simulink model "Milford"  (R2017a)
settings: Solver=FixedStepAuto  StartTime=0.0  StopTime=Cycle_End  FixedStep=0.01  MaxStep=0.01  RelTol=1e-3  EnableMultiTasking=on
PostLoadFcn:
  | , if any(exist('dsrtsu_mdlpostloadfcn', 'file') == [2, 3, 6]), try dsrtsu_mdlpostloadfcn('Execute', bdroot); catch fprintf('Error in PostLoadFcn (dsrtsu_mdlpostloadfcn) for model "%s":\n %s\n', bdroot, lasterr); end, end,
undefined symbols (not defined in the file): Actuators, APP1_OOR, APP2_OOR, APP_Mismatch, Brk_Flt, cal, ClutchEngag, DiscIntNeverNeededParam, eng, Engine, EngOverTemp, ENGTRQ_MSMCH_Degraded_CP, ENGTRQ_MSMCH_ErrCritical_CP, ENGTRQ_MSMCH_LimpHome_CP, EngTrqMismatch, ESSOverTemp, gb, Gearbox, KeyPos_Flt, lib_Actuators, lib_Sensors_2017a, lib_Transmission, Loss, LossCAN, MCUOverTemp, mot, MotDirMismatch, MotOverTemp, MotTrqMismatch, mph2kph, PRNDL_Flt, Ratio, RegenFault, Sensors, Spd, time, Transmission
libraries: simulink x110, powerlib_meascontrol x6, EC2_libraries x5, dspsigops x3, lib_Chassis x1, lib_DCDC x1, lib_Differential x1, lib_HVESS x1, lib_Engine x1, lib_OBC x1, Transmission_Validation x1, lib_Wheels x1
(part 2 of 9)

== system Milford/Fault Trigger /Component Diagnostics setting/Override  ESSOverTemp ==
  note: This subsystem is used to override the model value of a signal to a constant value
  note: Override Switch Subsystem
  In1 : Inport
  Constant : Constant  Value=0
  Multiport Switch : MultiPortSwitch  DataPortOrder=Zero-based contiguous  Inputs=2
  Signal Override Switch 0 = Use Model 1 = Use Constant : Constant  Value=ESSOverTemp_ON
  Out1 : Outport
  wires:
  Signal Override Switch 0 = Use Model 1 = Use Constant/1 -> Multiport Switch/1
  In1/1 -> Multiport Switch/2
  Multiport Switch/1 -> Out1/1
  Constant/1 -> Multiport Switch/3

== system Milford/Fault Trigger /Component Diagnostics setting/Override  EngOverTemp ==
  note: Override Switch Subsystem
  note: This subsystem is used to override the model value of a signal to a constant value
  In1 : Inport
  Constant : Constant  Value=0
  Multiport Switch : MultiPortSwitch  DataPortOrder=Zero-based contiguous  Inputs=2
  Signal Override Switch 0 = Use Model 1 = Use Constant : Constant  Value=EngOverTemp_ON
  Out1 : Outport
  wires:
  Constant/1 -> Multiport Switch/3
  Multiport Switch/1 -> Out1/1
  In1/1 -> Multiport Switch/2
  Signal Override Switch 0 = Use Model 1 = Use Constant/1 -> Multiport Switch/1

== system Milford/Fault Trigger /Component Diagnostics setting/Override  EngTrqMismatch ==
  note: This subsystem is used to override the model value of a signal to a constant value
  note: Override Switch Subsystem
  In1 : Inport
  Constant : Constant  Value=0
  Multiport Switch : MultiPortSwitch  DataPortOrder=Zero-based contiguous  Inputs=2
  Signal Override Switch 0 = Use Model 1 = Use Constant : Constant  Value=EngTrqMismatch_ON
  Out1 : Outport
  wires:
  Signal Override Switch 0 = Use Model 1 = Use Constant/1 -> Multiport Switch/1
  In1/1 -> Multiport Switch/2
  Multiport Switch/1 -> Out1/1
  Constant/1 -> Multiport Switch/3

== system Milford/Fault Trigger /Component Diagnostics setting/Override  LossCAN ==
  note: Override Switch Subsystem
  note: This subsystem is used to override the model value of a signal to a constant value
  In1 : Inport
  Constant : Constant  Value=0
  Multiport Switch : MultiPortSwitch  DataPortOrder=Zero-based contiguous  Inputs=2
  Signal Override Switch 0 = Use Model 1 = Use Constant : Constant  Value=LossCAN_ON
  Out1 : Outport
  wires:
  Constant/1 -> Multiport Switch/3
  Multiport Switch/1 -> Out1/1
  In1/1 -> Multiport Switch/2
  Signal Override Switch 0 = Use Model 1 = Use Constant/1 -> Multiport Switch/1

== system Milford/Fault Trigger /Component Diagnostics setting/Override  MCUOverTemp ==
  note: This subsystem is used to override the model value of a signal to a constant value
  note: Override Switch Subsystem
  In1 : Inport
  Constant : Constant  Value=0
  Multiport Switch : MultiPortSwitch  DataPortOrder=Zero-based contiguous  Inputs=2
  Signal Override Switch 0 = Use Model 1 = Use Constant : Constant  Value=MCUOverTemp_ON
  Out1 : Outport
  wires:
  Signal Override Switch 0 = Use Model 1 = Use Constant/1 -> Multiport Switch/1
  In1/1 -> Multiport Switch/2
  Multiport Switch/1 -> Out1/1
  Constant/1 -> Multiport Switch/3

== system Milford/Fault Trigger /Component Diagnostics setting/Override  MotDirMismatch ==
  note: Override Switch Subsystem
  note: This subsystem is used to override the model value of a signal to a constant value
  In1 : Inport
  Constant : Constant  Value=0
  Multiport Switch : MultiPortSwitch  DataPortOrder=Zero-based contiguous  Inputs=2
  Signal Override Switch 0 = Use Model 1 = Use Constant : Constant  Value=MotDirMismatch_ON
  Out1 : Outport
  wires:
  Constant/1 -> Multiport Switch/3
  Multiport Switch/1 -> Out1/1
  In1/1 -> Multiport Switch/2
  Signal Override Switch 0 = Use Model 1 = Use Constant/1 -> Multiport Switch/1

== system Milford/Fault Trigger /Component Diagnostics setting/Override  MotOverTemp ==
  note: Override Switch Subsystem
  note: This subsystem is used to override the model value of a signal to a constant value
  In1 : Inport
  Constant : Constant  Value=0
  Multiport Switch : MultiPortSwitch  DataPortOrder=Zero-based contiguous  Inputs=2
  Signal Override Switch 0 = Use Model 1 = Use Constant : Constant  Value=MotOverTemp_ON
  Out1 : Outport
  wires:
  Constant/1 -> Multiport Switch/3
  Multiport Switch/1 -> Out1/1
  In1/1 -> Multiport Switch/2
  Signal Override Switch 0 = Use Model 1 = Use Constant/1 -> Multiport Switch/1

== system Milford/Fault Trigger /Component Diagnostics setting/Override  MotTrqMismatch ==
  note: This subsystem is used to override the model value of a signal to a constant value
  note: Override Switch Subsystem
  In1 : Inport
  Constant : Constant  Value=0
  Multiport Switch : MultiPortSwitch  DataPortOrder=Zero-based contiguous  Inputs=2
  Signal Override Switch 0 = Use Model 1 = Use Constant : Constant  Value=MotTrqMismatch_ON
  Out1 : Outport
  wires:
  Signal Override Switch 0 = Use Model 1 = Use Constant/1 -> Multiport Switch/1
  In1/1 -> Multiport Switch/2
  Multiport Switch/1 -> Out1/1
  Constant/1 -> Multiport Switch/3

== system Milford/Fault Trigger /Driver Interface Diagnostics setting/Override  APP1_OOR ==
  note: Signal Override Switch
      | 0 = Use Model
      | 1 = Use Constant
  note: Override Switch Subsystem
  note: This subsystem is used to override the model value of a signal to a constant value
  In1 : Inport
  APP1_OOR_ON : Constant  Value=APP1_OOR_ON
  Constant : Constant  Value=0
  Multiport Switch : MultiPortSwitch  DataPortOrder=Zero-based contiguous  Inputs=2
  Out1 : Outport
  wires:
  Constant/1 -> Multiport Switch/3
  Multiport Switch/1 -> Out1/1
  In1/1 -> Multiport Switch/2
  APP1_OOR_ON/1 -> Multiport Switch/1

== system Milford/Fault Trigger /Driver Interface Diagnostics setting/Override  APP2_OOR ==
  note: Signal Override Switch
      | 0 = Use Model
      | 1 = Use Constant
  note: This subsystem is used to override the model value of a signal to a constant value
  note: Override Switch Subsystem
  In1 : Inport
  APP2_OOR_ON : Constant  Value=APP2_OOR_ON
  Constant : Constant  Value=0
  Multiport Switch : MultiPortSwitch  DataPortOrder=Zero-based contiguous  Inputs=2
  Out1 : Outport
  wires:
  APP2_OOR_ON/1 -> Multiport Switch/1
  In1/1 -> Multiport Switch/2
  Multiport Switch/1 -> Out1/1
  Constant/1 -> Multiport Switch/3

== system Milford/Fault Trigger /Driver Interface Diagnostics setting/Override  APP_Mismatch ==
  note: Signal Override Switch
      | 0 = Use Model
      | 1 = Use Constant
  note: Override Switch Subsystem
  note: This subsystem is used to override the model value of a signal to a constant value
  In1 : Inport
  APP_Mismatch_Override : Constant  Value=Mismatch_APP_ON
  Constant : Constant  Value=0
  Multiport Switch : MultiPortSwitch  DataPortOrder=Zero-based contiguous  Inputs=2
  Out1 : Outport
  wires:
  Constant/1 -> Multiport Switch/3
  Multiport Switch/1 -> Out1/1
  In1/1 -> Multiport Switch/2
  APP_Mismatch_Override/1 -> Multiport Switch/1

== system Milford/Fault Trigger /Driver Interface Diagnostics setting/Override  BPP_Flt ==
  note: Signal Override Switch
      | 0 = Use Model
      | 1 = Use Constant
  note: This subsystem is used to override the model value of a signal to a constant value
  note: Override Switch Subsystem
  In1 : Inport
  Brk_Flt_ON : Constant  Value=Brk_Flt_ON
  Constant : Constant  Value=0
  Multiport Switch : MultiPortSwitch  DataPortOrder=Zero-based contiguous  Inputs=2
  Out1 : Outport
  wires:
  Brk_Flt_ON/1 -> Multiport Switch/1
  In1/1 -> Multiport Switch/2
  Multiport Switch/1 -> Out1/1
  Constant/1 -> Multiport Switch/3

== system Milford/Fault Trigger /Driver Interface Diagnostics setting/Override  KeyPos_Flt ==
  note: Signal Override Switch
      | 0 = Use Model
      | 1 = Use Constant
  note: Override Switch Subsystem
  note: This subsystem is used to override the model value of a signal to a constant value
  In1 : Inport
  Constant : Constant  Value=0
  KeyPos_Flt_ON : Constant  Value=KeyPos_Flt_ON
  Multiport Switch : MultiPortSwitch  DataPortOrder=Zero-based contiguous  Inputs=2
  Out1 : Outport
  wires:
  Constant/1 -> Multiport Switch/3
  Multiport Switch/1 -> Out1/1
  In1/1 -> Multiport Switch/2
  KeyPos_Flt_ON/1 -> Multiport Switch/1

== system Milford/Fault Trigger /Driver Interface Diagnostics setting/Override  PRNDL_Flt ==
  note: Signal Override Switch
      | 0 = Use Model
      | 1 = Use Constant
  note: This subsystem is used to override the model value of a signal to a constant value
  note: Override Switch Subsystem
  In1 : Inport
  Constant : Constant  Value=0
  Multiport Switch : MultiPortSwitch  DataPortOrder=Zero-based contiguous  Inputs=2
  PRNDL_Flt_ON : Constant  Value=PRNDL_Flt_ON
  Out1 : Outport
  wires:
  PRNDL_Flt_ON/1 -> Multiport Switch/1
  In1/1 -> Multiport Switch/2
  Multiport Switch/1 -> Out1/1
  Constant/1 -> Multiport Switch/3

== system Milford/Sensors/CAN/EBCAN ==
  In1 : Inport
  BMS_Antrieb : Subsystem
  Bus Creator : BusCreator  Inputs=3
  Bus Selector : BusSelector  OutputSignals=ECM_CAN,BMS_CAN.BMS_Hybrid
  CCM : Subsystem
  ECM : Subsystem
  Out1 : Outport
  wires:
  Bus Selector/2 -> BMS_Antrieb/1(In1), CCM/1(In1)  "<BMS_Hybrid>"
  Bus Selector/1 -> ECM/1(In1)  "<ECM_CAN>"
  In1/1 -> Bus Selector/1
  CCM/1(Out1) -> Bus Creator/3  "from_CCM"
  Bus Creator/1 -> Out1/1
  BMS_Antrieb/1(Out1) -> Bus Creator/2  "from_BMSAntrieb"
  ECM/1(Out1) -> Bus Creator/1  "from_ECM"

== system Milford/Sensors/CAN/HV_CAN ==
  In1 : Inport
  BMS_Hybrid : Subsystem
  Bus Creator : BusCreator  Inputs=2
  Bus Selector : BusSelector  OutputSignals=BMS_CAN.BMS_Plugin,OBC_CAN
  OBC : Subsystem
  Out1 : Outport
  wires:
  Bus Selector/2 -> OBC/1(In1)  "<OBC_CAN>"
  Bus Selector/1 -> BMS_Hybrid/1(In1)  "<BMS_Plugin>"
  In1/1 -> Bus Selector/1
  Bus Creator/1 -> Out1/1
  OBC/1(Out1) -> Bus Creator/2  "from_OBC"
  BMS_Hybrid/1(Out1) -> Bus Creator/1  "from_BMSHybrid"

== system Milford/Sensors/CAN/VEH_CAN ==
  In1 : Inport
  BCM : Subsystem
  Bus Creator : BusCreator  Inputs=4
  Bus Selector : BusSelector  OutputSignals=TCM_CAN,BCM_CAN
  EBCM : Subsystem  Commented=on
  Ground : Ground  Commented=on
  Ground1 : Ground  Commented=on
  ICCM : Subsystem  Commented=on
  TCM : Subsystem
  Out1 : Outport
  wires:
  Ground/1 -> EBCM/1(In1)  "<EBCM>"
  Ground1/1 -> ICCM/1(In1)  "<ONSTAR>"
  Bus Selector/2 -> BCM/1(In1)  "<BCM_CAN>"
  Bus Selector/1 -> TCM/1(In1)  "<TCM_CAN>"
  Bus Creator/1 -> Out1/1
  EBCM/1(Out1) -> Bus Creator/4  "from_EBCM"
  ICCM/1(Out1) -> Bus Creator/3  "from_ICCM"
  BCM/1(Out1) -> Bus Creator/2  "from_BCM"
  TCM/1(Out1) -> Bus Creator/1  "from_TCM"
  In1/1 -> Bus Selector/1

== system Milford/Actuators/CAN/EBCAN/ISO_Hybrid_01_Req ==
  In1 : Inport
  Bus Creator : BusCreator  Inputs=1
  Bus Selector : BusSelector  OutputSignals=ISO_Hybrid_01_Req_Data_byte_3
  Data Type Conversion : DataTypeConversion
  Out1 : Outport
  wires:
  In1/1 -> Bus Selector/1
  Data Type Conversion/1 -> Bus Creator/1  "ISO_Hybrid_01_Req_Data_4"
  Bus Creator/1 -> Out1/1  "ISO_Hybrid_01_Req"
  Bus Selector/1 -> Data Type Conversion/1  "<ISO_Hybrid_01_Req_Data_byte_3>"

== system Milford/Actuators/CAN/EBCAN/PPEI_Platform_General_Status ==
  In1 : Inport
  Bus Creator : BusCreator  Inputs=1
  Data Type Conversion : DataTypeConversion
  Out1 : Outport
  wires:
  Bus Creator/1 -> Out1/1  "PPEI_Platform_General_Status"
  Data Type Conversion/1 -> Bus Creator/1  "SysPwrMd"
  In1/1 -> Data Type Conversion/1

== system Milford/Actuators/CAN/EBCAN/PPEI_Trans_General_Status_2 ==
  In1 : Inport
  Bus Creator : BusCreator  Inputs=1
  Data Type Conversion : DataTypeConversion
  Out1 : Outport
  wires:
  In1/1 -> Data Type Conversion/1
  Data Type Conversion/1 -> Bus Creator/1  "TrnsShftLvrPos"
  Bus Creator/1 -> Out1/1  "PPEI_Trans_General_Status_2"

== system Milford/Actuators/CAN/VEH_CAN/BCM ==
  In1 : Inport
  Bus Creator : BusCreator  Inputs=1
  Bus Selector : BusSelector  OutputSignals=Controls.powerMode
  Out1 : Outport
  wires:
  In1/1 -> Bus Selector/1
  Bus Selector/1 -> Bus Creator/1  "<powerMode>"
  Bus Creator/1 -> Out1/1

== system Milford/Actuators/CAN/VEH_CAN/EBCM ==
  In1 : Inport
  Out1 : Outport
  wires:
  In1/1 -> Out1/1

== system Milford/Actuators/CAN/VEH_CAN/ICCM ==
  In1 : Inport
  Out1 : Outport
  wires:
  In1/1 -> Out1/1

== system Milford/Camaro Plant Model/Calculate MPGe/Calculate MPGe/Calculate Fuel Economy ==
  Kph : Inport
  Fuel Flow g/s : Inport  Port=2
  1 : Constant
  Cumulative Distance Km : DiscreteIntegrator  InitialCondition=eps  SampleTime=-1  ICPrevOutput=DiscIntNeverNeededParam  ICPrevScaledInput=DiscIntNeverNeededParam
  Cumulative Gal : DiscreteIntegrator  InitialCondition=eps  SampleTime=-1  ICPrevOutput=DiscIntNeverNeededParam  ICPrevScaledInput=DiscIntNeverNeededParam
  Cumulative L : DiscreteIntegrator  InitialCondition=eps  SampleTime=-1  ICPrevOutput=DiscIntNeverNeededParam  ICPrevScaledInput=DiscIntNeverNeededParam
  Divide : Product  Inputs=*/
  Divide1 : Product  Inputs=*/
  Gasoline Density Kg/L : Constant  Value=0.7871
  Gasoline Density Kg/L1 : Constant  Value=0.7871
  Km to miles : Gain  Gain=1/1.609344
  Kph to Kps : Gain  Gain=1/3600
  L/Km : Product  Inputs=/*
  L/Km to L/100Km : Gain  Gain=100
  Product : Product
  To Workspace : ToWorkspace  VariableName=Fuel_mass  SampleTime=-1
  g : Gain  Gain=1000
  g/s to Kg/s : Gain  Gain=0.001
  km/l : Product  Inputs=/*
  m^3 to gal : Gain  Gain=264.172
  Liter/100Km : Outport
  Km/Liter : Outport  Port=2
  MPG : Outport  Port=3
  Fuel Used (L) : Outport  Port=4
  wires:
  km/l/1 -> Km/Liter/1
  1/1 -> km/l/2
  Divide1/1 -> MPG/1
  L/Km to L/100Km/1 -> Liter/100Km/1
  Fuel Flow g/s/1 -> g/s to Kg/s/1
  Kph/1 -> Kph to Kps/1
  Cumulative Gal/1 -> Divide1/2
  Km to miles/1 -> Divide1/1
  L/Km/1 -> km/l/1, L/Km to L/100Km/1
  Cumulative Distance Km/1 -> Km to miles/1, L/Km/1
  Kph to Kps/1 -> Cumulative Distance Km/1
  m^3 to gal/1 -> Cumulative Gal/1
  Divide/1 -> Cumulative L/1, m^3 to gal/1
  Gasoline Density Kg/L/1 -> Divide/2
  g/s to Kg/s/1 -> Divide/1
  Cumulative L/1 -> L/Km/2, Product/1, Fuel Used (L)/1
  Gasoline Density Kg/L1/1 -> Product/2
  Product/1 -> g/1
  g/1 -> To Workspace/1

== system Milford/Camaro Plant Model/Scopes/AxlTrq_to_EngTrq2/Ratio Filter ==
  Ratio : Inport
  Abs : Abs
  Compare To Zero : simulink/Logic and Bit Operations/Compare To Zero  relop===  OutDataTypeStr=boolean
  Constant : Constant  Value=cal.Time.TrnsOvrllEstTrqRatioSwitch
  Mature_Delay : EC2_libraries/Mature_Delay
      settings: SourceProductName=The database C:\Users\vrajm\AppData\Roaming\MathWorks\MATLAB\R2017b\slblocks_master.db is locked, or a table in the database is locked. (database is locked)
  Memory1 : Memory  X0=1
  Switch1 : Switch  Threshold=1
  Switch2 : Switch  Threshold=1
  Filtered_Ratio : Outport
  wires:
  Ratio/1 -> Compare To Zero/1, Abs/1
  Compare To Zero/1 -> Mature_Delay/1, Switch2/2
  Abs/1 -> Switch1/1, Switch2/3
  Switch1/1 -> Switch2/1
  Constant/1 -> Mature_Delay/2
  Mature_Delay/1 -> Switch1/2
  Memory1/1 -> Switch1/3
  Switch2/1 -> Filtered_Ratio/1, Memory1/1  "gear_ratio"

== system Milford/Camaro Plant Model/Scopes/AxlTrq_to_MtrTrq2/Ratio Filter ==
  Ratio : Inport
  Abs : Abs
  Compare To Zero : simulink/Logic and Bit Operations/Compare To Zero  relop===  OutDataTypeStr=boolean
  Constant : Constant  Value=cal.Time.TrnsOvrllEstTrqRatioSwitch
  Mature_Delay : EC2_libraries/Mature_Delay
      settings: SourceProductName=The database C:\Users\vrajm\AppData\Roaming\MathWorks\MATLAB\R2017b\slblocks_master.db is locked, or a table in the database is locked. (database is locked)
  Memory1 : Memory  X0=1
  Switch1 : Switch  Threshold=1
  Switch2 : Switch  Threshold=1
  Filtered_Ratio : Outport
  wires:
  Ratio/1 -> Compare To Zero/1, Abs/1
  Compare To Zero/1 -> Mature_Delay/1, Switch2/2
  Abs/1 -> Switch1/1, Switch2/3
  Switch1/1 -> Switch2/1
  Constant/1 -> Mature_Delay/2
  Mature_Delay/1 -> Switch1/2
  Memory1/1 -> Switch1/3
  Switch2/1 -> Filtered_Ratio/1, Memory1/1  "gear_ratio"

== system Milford/Camaro Plant Model/Transmission/Inputs/Analog_fromHCU ==
  Outputs : Outport
  wires:
  [Analog] -> Outputs/1

== system Milford/Camaro Plant Model/Transmission/Inputs/CAN_fromHCU ==
  Outputs : Outport
  wires:
  [HCU_to_VEH_CAN] -> Outputs/1

== system Milford/Camaro Plant Model/Transmission/Inputs/Digital_fromHCU ==
  Outputs : Outport
  wires:
  [Digital] -> Outputs/1

== system Milford/Camaro Plant Model/Transmission/Soft TCM/6L45 Logic/Gearbox_Control.Shift_Schedule.PlotShiftSchedule ==
  f : TriggerPort  TriggerType=function-call  VariantControl=Variant
      settings: CopyFcn=Stateflow.SLINSF.SimulinkMan.removeBlockPreDeleteFcn  PreDeleteFcn=Stateflow.SLINSF.SimulinkMan.unsafePredeleteFcn
  Subsystem : Subsystem
      settings: OpenFcn=|
      | figure;
      | PlotGearShiftSchedule(Gearbox.L45.PedalPositions,Gearbox.L45.UpShiftSpeeds,Gearbox.L45.DownShiftSpeeds,'6L45')
      mask Display: disp('Plot')

== system Milford/Camaro Plant Model/Transmission/Soft TCM/6L45 Logic/Gearbox_Control.Shift_Schedule.calc_down ==
  Gear : Inport
  APP : Inport  Port=2
  f : TriggerPort  TriggerType=function-call  VariantControl=Variant
      settings: CopyFcn=Stateflow.SLINSF.SimulinkMan.removeBlockPreDeleteFcn  PreDeleteFcn=Stateflow.SLINSF.SimulinkMan.unsafePredeleteFcn
  Calculate Downshift Threshold : Lookup2D  RowIndex=gb.ctrl.dmd.init.gear_dnshift.idx1_lin_accel  ColumnIndex=[2,3,4,5,6,7,8]  Table=gb.ctrl.dmd.init.gear_dnshift.map'  LookUpMeth=Interpolation-Use End Values
  down_th : Outport
  wires:
  Calculate Downshift Threshold/1 -> down_th/1
  Gear/1 -> Calculate Downshift Threshold/2
  APP/1 -> Calculate Downshift Threshold/1

== system Milford/Camaro Plant Model/Transmission/Soft TCM/6L45 Logic/Gearbox_Control.Shift_Schedule.calc_up ==
  Gear : Inport
  APP : Inport  Port=2
  f : TriggerPort  TriggerType=function-call  VariantControl=Variant
      settings: CopyFcn=Stateflow.SLINSF.SimulinkMan.removeBlockPreDeleteFcn  PreDeleteFcn=Stateflow.SLINSF.SimulinkMan.unsafePredeleteFcn
  Calculate Upshift Threshold : Lookup2D  RowIndex=gb.ctrl.dmd.init.gear_upshift.idx1_lin_accel  ColumnIndex=[1,2,3,4,5,6,7]  Table=gb.ctrl.dmd.init.gear_upshift.map'  LookUpMeth=Interpolation-Use End Values
  up_th : Outport
  wires:
  Calculate Upshift Threshold/1 -> up_th/1
  APP/1 -> Calculate Upshift Threshold/1
  Gear/1 -> Calculate Upshift Threshold/2

== system Milford/Camaro Plant Model/Transmission/Soft TCM/6L45 Logic/Torque_Converter_Control.calc_lockup ==
  Gear : Inport
  APP : Inport  Port=2
  f : TriggerPort  TriggerType=function-call  VariantControl=Variant
      settings: CopyFcn=Stateflow.SLINSF.SimulinkMan.removeBlockPreDeleteFcn  PreDeleteFcn=Stateflow.SLINSF.SimulinkMan.unsafePredeleteFcn
  Calculate Lockup Threshold : Lookup2D  RowIndex=cpl.ctrl.init.trqconv_lockup.idx1_lin_accel  ColumnIndex=cpl.ctrl.init.trqconv_lockup.idx2_gear  Table=cpl.ctrl.init.trqconv_lockup.map  LookUpMeth=Interpolation-Use End Values
  lockup_th : Outport
  wires:
  Calculate Lockup Threshold/1 -> lockup_th/1
  APP/1 -> Calculate Lockup Threshold/1
  Gear/1 -> Calculate Lockup Threshold/2

== system Milford/Camaro Plant Model/Transmission/Soft TCM/6L45 Logic/Torque_Converter_Control.calc_unlock ==
  Gear : Inport
  APP : Inport  Port=2
  f : TriggerPort  TriggerType=function-call  VariantControl=Variant
      settings: CopyFcn=Stateflow.SLINSF.SimulinkMan.removeBlockPreDeleteFcn  PreDeleteFcn=Stateflow.SLINSF.SimulinkMan.unsafePredeleteFcn
  Calculate Unlock Threshold : Lookup2D  RowIndex=cpl.ctrl.init.trqconv_unlock.idx1_lin_accel  ColumnIndex=cpl.ctrl.init.trqconv_unlock.idx2_gear  Table=cpl.ctrl.init.trqconv_unlock.map  LookUpMeth=Interpolation-Use End Values
  unlock_th : Outport
  wires:
  Calculate Unlock Threshold/1 -> unlock_th/1
  APP/1 -> Calculate Unlock Threshold/1
  Gear/1 -> Calculate Unlock Threshold/2

== system Milford/Camaro Plant Model/Transmission/Transmission Plant/ Actuators ==
  In1 : Inport
  Bus Selector : BusSelector  OutputSignals=TransEstGear,LockupCmd
  Out2 : Outport
  Out5 : Outport  Port=2
  wires:
  In1/1 -> Bus Selector/1
  Bus Selector/1 -> Out2/1  "<TransEstGear>"
  Bus Selector/2 -> Out5/1  "<LockupCmd>"

== system Milford/Camaro Plant Model/Transmission/Transmission Plant/Gearbox ==
  TransEstGear : Inport
  gb_trq_in gb_inertia_in : Inport  Port=2
  gb_spd_out : Inport  Port=3
  Bus Creator : BusCreator  Inputs=2
  Bus Selector : BusSelector  OutputSignals=tc_trq_out,tc_inertia_out
  Engine Inertia : Constant  Value=Engine.Inertia
  Gear : Lookup  InputValues=gb.plant.init.gear.idx1_shifter  Table=gb.plant.init.gear.idx2_gear  LookUpMeth=Interpolation-Use End Values  OutDataTypeStr=double  SaturateOnIntegerOverflow=on
  Inertia Calculation : Subsystem
  Memory : Memory
  Speed Calculation : Subsystem
  Subsystem : Subsystem
  To Workspace : ToWorkspace  VariableName=TOSS  SampleTime=-1
  Torque calculation : Subsystem
  gear ratio table : Lookup  InputValues=gb.plant.init.ratio.idx1_gear  Table=gb.plant.init.ratio.map  LookUpMeth=Interpolation-Use End Values  SaturateOnIntegerOverflow=on
  gb_trq_out gb_inertia_out : Outport
  gb_spd_in : Outport  Port=2
  tag scope: gb_gear=global, gb_inertia_in=global, gb_inertia_out=global, gb_spd_in=global, gb_spd_out=global, gb_trq_in=global, gb_trq_out=global, gb_trq_ratio=global
  wires:
  Bus Selector/2 -> Inertia Calculation/1(Inertia_in), Speed Calculation/4(Inertia Input)  "<tc_inertia_out>"
  Engine Inertia/1 -> [gb_inertia_in]
  Subsystem/1(Out1) -> [gb_trq_out], Bus Creator/1  "gb_trq_out"
  Torque calculation/1(torque_out) -> Subsystem/1(In1), Subsystem/2(In2)  "gb_trq_out"
  Memory/1 -> Gear/1
  gear ratio table/1 -> [gb_trq_ratio]
  Bus Creator/1 -> gb_trq_out gb_inertia_out/1
  Inertia Calculation/1(Inertia) -> Bus Creator/2, [gb_inertia_out]  "gb_inertia_out"
  Speed Calculation/1(Speed) -> gb_spd_in/1, [gb_spd_in]
  gb_trq_in gb_inertia_in/1 -> Bus Selector/1
  gb_spd_out/1 -> Speed Calculation/2(spd out), [gb_spd_out], To Workspace/1, Torque calculation/1(speed out)
  Gear/1 -> Torque calculation/2(gear number), Inertia Calculation/2(gear number), gear ratio table/1, [gb_gear], Speed Calculation/1(gear number)
  Bus Selector/1 -> Torque calculation/3(" input torque"), Speed Calculation/3(torque input), [gb_trq_in]  "<tc_trq_out>"
  TransEstGear/1 -> Memory/1

== system Milford/Camaro Plant Model/Transmission/Transmission Plant/Sensors ==
  In2 : Inport
  In3 : Inport  Port=2
  In4 : Inport  Port=3
  In5 : Inport  Port=4
  In6 : Inport  Port=5
  In7 : Inport  Port=6
  In1 : Inport  Port=7
  Bus Creator : BusCreator  Inputs=7
  Out1 : Outport
  wires:
  In1/1 -> Bus Creator/7  "gb_trq_ratio"
  Bus Creator/1 -> Out1/1
  In2/1 -> Bus Creator/1  "impeller_spd_rads"
  In4/1 -> Bus Creator/3  "tc_trq_in"
  In5/1 -> Bus Creator/4  "tc_trq_out"
  In3/1 -> Bus Creator/2  "turbine_spd_rads"
  In6/1 -> Bus Creator/5  "TrnsOutShftAngVel"
  In7/1 -> Bus Creator/6  "TrnsOutShftTrq"

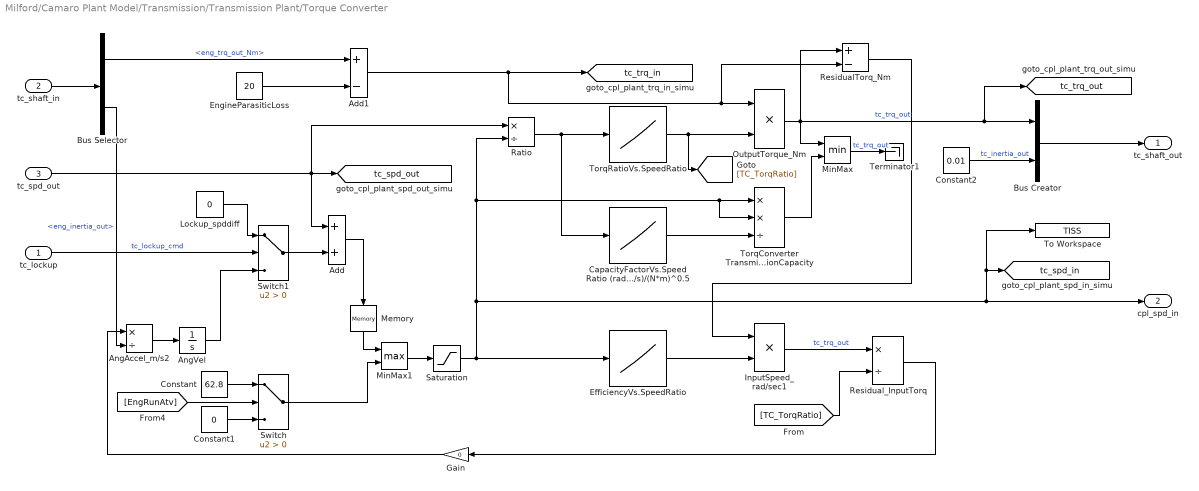
== system Milford/Camaro Plant Model/Transmission/Transmission Plant/Torque Converter ==
  tc_lockup : Inport
  tc_shaft_in : Inport  Port=2
  tc_spd_out : Inport  Port=3
  Add : Sum
  Add1 : Sum  Inputs=+-
  AngAccel_m/s2 : Product  Inputs=*/
  AngVel : Integrator
  Bus Creator : BusCreator  Inputs=2
  Bus Selector : BusSelector  OutputSignals=eng_trq_out_Nm,eng_inertia_out
  CapacityFactorVs.SpeedRatio (rad/s)/(N*m)^0.5 : Lookup_n-D  NumberOfTableDimensions=1  BreakpointsForDimension1=[0 0.50 0.60 0.70 0.80 0.87 0.92 0.94 0.96 0.97]  Table=[12.2938 12.8588 13.1452 13.6285 14.6163 16.2675 19.3503 22.1046 29.9986 50.00]  InternalRulePriority=Speed  RndMeth=Simplest  InputSameDT=on
  Constant : Constant  Value=62.8
  Constant1 : Constant  Value=0
  Constant2 : Constant  Value=0.01
  EfficiencyVs.SpeedRatio : Lookup_n-D  NumberOfTableDimensions=1  BreakpointsForDimension1=[0 0.25 0.50 0.60 0.70 0.80 0.87 0.92 0.94 0.96 0.97 1.0]  Table="[0.10 0.50 0.70 0.8 0.8 0.80  0.85 0.87 0.91 0.95 0.96 0.96]"  InternalRulePriority=Speed  RndMeth=Simplest  InputSameDT=on
  EngineParasiticLoss : Constant  Value=20
  Gain : Gain  Gain=0
  InputSpeed_rad/sec1 : Product  Inputs=**
  Lockup_spddiff : Constant  Value=0
  Memory : Memory  X0=1
  MinMax : MinMax  Inputs=2
  MinMax1 : MinMax  Function=max  Inputs=2
  OutputTorque_Nm : Product  Inputs=**
  Ratio : Product  Inputs=*/
  ResidualTorq_Nm : Sum  Inputs=+-
  Residual_InputTorq : Product  Inputs=*/
  Saturation : Saturate  UpperLimit=1100  LowerLimit=1
  Switch : Switch  Criteria=u2 > Threshold
  Switch1 : Switch  Criteria=u2 > Threshold
  Terminator1 : Terminator
  To Workspace : ToWorkspace  VariableName=TISS  SampleTime=-1
  TorqConverter TransmissionCapacity : Product  Inputs=**/
  TorqRatioVs.SpeedRatio : Lookup_n-D  NumberOfTableDimensions=1  BreakpointsForDimension1=[0 0.50 0.60 0.70 0.80 0.87 0.92 0.94 0.96 0.97]  Table=[2.2320 1.5462 1.4058 1.2746 1.1528 1.0732 1.0192 0.9983 0.9983 0.9983]  InternalRulePriority=Speed  RndMeth=Simplest  InputSameDT=on
  tc_shaft_out : Outport
  cpl_spd_in : Outport  Port=2
  tag scope: tc_spd_in=global, tc_spd_out=global, tc_trq_in=global, tc_trq_out=global
  wires:
  Lockup_spddiff/1 -> Switch1/1
  Switch1/1 -> Add/2
  Bus Selector/1 -> Add1/1  "<eng_trq_out_Nm>"
  Constant1/1 -> Switch/3
  Constant/1 -> Switch/1
  [EngRunAtv] -> Switch/2
  Switch/1 -> MinMax1/2
  MinMax1/1 -> Saturation/1
  Gain/1 -> AngAccel_m/s2/1
  Add/1 -> Memory/1
  tc_spd_out/1 -> Add/1, [tc_spd_out], Ratio/1
  MinMax/1 -> Terminator1/1  "tc_trq_out"
  OutputTorque_Nm/1 -> MinMax/1, [tc_trq_out], Bus Creator/1, ResidualTorq_Nm/1  "tc_trq_out"
  Residual_InputTorq/1 -> Gain/1
  EngineParasiticLoss/1 -> Add1/2
  Memory/1 -> MinMax1/1
  AngVel/1 -> Switch1/3
  AngAccel_m/s2/1 -> AngVel/1
  InputSpeed_rad/sec1/1 -> Residual_InputTorq/1  "tc_trq_out"
  ResidualTorq_Nm/1 -> InputSpeed_rad/sec1/1
  [TC_TorqRatio] -> Residual_InputTorq/2
  TorqConverter TransmissionCapacity/1 -> MinMax/2
  EfficiencyVs.SpeedRatio/1 -> InputSpeed_rad/sec1/2
  Saturation/1 -> EfficiencyVs.SpeedRatio/1, cpl_spd_in/1, To Workspace/1, [tc_spd_in], TorqConverter TransmissionCapacity/1, TorqConverter TransmissionCapacity/2, Ratio/2
  Ratio/1 -> TorqRatioVs.SpeedRatio/1, CapacityFactorVs.SpeedRatio (rad/s)/(N*m)^0.5/1
  CapacityFactorVs.SpeedRatio (rad/s)/(N*m)^0.5/1 -> TorqConverter TransmissionCapacity/3
  TorqRatioVs.SpeedRatio/1 -> [TC_TorqRatio], OutputTorque_Nm/2
  tc_lockup/1 -> Switch1/2  "tc_lockup_cmd"
  Bus Selector/2 -> AngAccel_m/s2/2  "<eng_inertia_out>"
  Bus Creator/1 -> tc_shaft_out/1
  tc_shaft_in/1 -> Bus Selector/1
  Constant2/1 -> Bus Creator/2  "tc_inertia_out"
  Add1/1 -> OutputTorque_Nm/1, ResidualTorq_Nm/2, [tc_trq_in]

== system Milford/Controller_with_Transmission_Manager1/HSC/Camaro Fault Detection/Component Diagnostic ==
  note: Component Diagnostics
  note: Component Status Setting Rule
      | xxx_CompStatus could be 0, 1, 2 or 3
      | 0: component needs to be offline
      | 1: component needs torque plant to deliver creep torque
      | 2: component needs torque plant to limit maximum torque delivery
      | 3: component needs torque plant to operate normally
  SignalDiag : Inport
  Bus Creator : BusCreator  Inputs=6
  Driver Input Diagnostic : Subsystem
  ESS Component Diagnostic : Subsystem
  Engine Component Diagnostic : Subsystem
  Override Driver Status : Subsystem
  Override ESS Status : Subsystem
  Override Engine Status : Subsystem
  Override TCM Status : Subsystem
  Transmission Component Diagnostic : Subsystem
  CompDiag : Outport
  wires:
  Engine Component Diagnostic/2(Out2) -> Bus Creator/4  "EngTrqMismchType"
  Override Driver Status/1(Out1) -> Bus Creator/1  "Driver_Input_Status"
  Override TCM Status/1(Out1) -> Bus Creator/5  "TCM_Status"
  Override Engine Status/1(Out1) -> Bus Creator/3  "ECM_Status"
  Override ESS Status/1(Out1) -> Bus Creator/2  "BMS_Status"
  Transmission Component Diagnostic/1(Out1) -> Override TCM Status/1(In1)  "TCM_CompDiag"
  Engine Component Diagnostic/1(Out1) -> Override Engine Status/1(In1)  "ECM_CompDiag"
  ESS Component Diagnostic/1(Out1) -> Override ESS Status/1(In1)  "ESS_CompDiag"
  Driver Input Diagnostic/1(Out1) -> Override Driver Status/1(In1)  "Diver_CompDiag"
  Bus Creator/1 -> CompDiag/1
  SignalDiag/1 -> Driver Input Diagnostic/1(In1), ESS Component Diagnostic/1(In1), Bus Creator/6, Transmission Component Diagnostic/1(In1), Engine Component Diagnostic/1(In1)  "RawSig"

== system Milford/Controller_with_Transmission_Manager1/HSC/Camaro Fault Detection/Input Conversions ==
  note: These subsystems convert variable types to match those used in the
      | supervisor. In addition, override switches installed on each signal can
      | be used to manually override and signal for testing purposes
  note: Input Conversions and Override Switches
  RawSig : Inport
  BMS_Conversions : Subsystem
  Bus Creator : BusCreator  Inputs=5
  DriverInput_Conversions : Subsystem
  ECM_Conversions : Subsystem
  TCM_Conversions : Subsystem
  VehSig : Outport
  wires:
  TCM_Conversions/1(Out1) -> Bus Creator/4
  ECM_Conversions/1(Out1) -> Bus Creator/3
  RawSig/1 -> BMS_Conversions/1(In1), ECM_Conversions/1(In1), TCM_Conversions/1(In1), Bus Creator/5, DriverInput_Conversions/1(In1)  "RawSig"
  BMS_Conversions/1(Out1) -> Bus Creator/2
  Bus Creator/1 -> VehSig/1  "InputConvAndOvrd"
  DriverInput_Conversions/1(Out1) -> Bus Creator/1

== system Milford/Controller_with_Transmission_Manager1/HSC/Camaro Fault Detection/Signal Diagnostic ==
  note: Signal Diagnostics
  note: These subsystems evaluate each signal for proper value range and other checks
  VehSig : Inport
  Bus Creator : BusCreator  Inputs=5
  Driver Signal Diagnostic : Subsystem
  ESS Signal Diagnostic : Subsystem
  Engine Signal Diagnostic : Subsystem
  Subsystem1 : Subsystem
      mask Display: fprintf('Signal Naming Rule')
  Transmission Signal Diagnostic : Subsystem
  SignalDiag : Outport
  wires:
  Bus Creator/1 -> SignalDiag/1  "SignalDiag"
  Transmission Signal Diagnostic/1(Out2) -> Bus Creator/4  "Transmission_SigDiag"
  Engine Signal Diagnostic/1(Engine_SigDiag) -> Bus Creator/3  "Engine_SigDiag"
  ESS Signal Diagnostic/1(ESS_SigDiag) -> Bus Creator/2  "ESS_SigDiag"
  Driver Signal Diagnostic/1(Driver_SigDiag) -> Bus Creator/1  "Driver_SigDiag"
  VehSig/1 -> Transmission Signal Diagnostic/1(Sensors1), Bus Creator/5, Engine Signal Diagnostic/1(Sensors1), Driver Signal Diagnostic/1(Sensors1), ESS Signal Diagnostic/1(Sensors1)

== system Milford/Controller_with_Transmission_Manager1/HSC/Driver_Requests/APP_BPP to DrvIntndAxlTrq2 ==
  note: Note:Driver requested Axle Torque Calculation
  note: $Author: fy6949 $
      | $Rev: 577 $
      | $Date: 2017-1-19 08:53:15 -0500  $
  Sensors : Inport
  Diag : Inport  Port=2
  Controls : Inport  Port=3
  Bus Selector : BusSelector  OutputSignals=from_Analog.Driver_APP1,from_CAN.fromVEH_CAN.from_BCM.BrkPdlPos,from_CAN.fromEBCAN.from_ECM.VehSpdAvgDrvn,from_CAN.fromVEH_CAN.from_TCM.TrnGrRat
  Bus Selector1 : BusSelector  OutputSignals=CompSig.RawSig.Driver_SigDiag.Drv_APP_Agree
  Bus Selector2 : BusSelector  OutputSignals=mode
  Constant : Constant  Value=0
  Post Driver Intnded Axle Torque : Subsystem
  Terminator : Terminator
  Terminator1 : Terminator
  IntndAxlTrq : Outport
  wires:
  Sensors/1 -> Bus Selector/1
  Controls/1 -> Bus Selector2/1
  Post Driver Intnded Axle Torque/1(IntndAxlTrq) -> IntndAxlTrq/1
  Bus Selector/2 -> Post Driver Intnded Axle Torque/2(BPP)  "<BrkPdlPos>"
  Bus Selector/3 -> Post Driver Intnded Axle Torque/3(VehicleSpeed)  "<VehSpdAvgDrvn>"
  Bus Selector/4 -> Post Driver Intnded Axle Torque/4(TransGearRatio)  "<TrnGrRat>"
  Bus Selector/1 -> Post Driver Intnded Axle Torque/1(APP)  "<Driver_APP1>"
  Post Driver Intnded Axle Torque/2(BrkIntndAxlTrq) -> Terminator/1
  Diag/1 -> Bus Selector1/1
  Bus Selector1/1 -> Terminator1/1  "<Drv_APP_Agree>"
  Bus Selector2/1 -> Post Driver Intnded Axle Torque/5(Mode)  "<mode>"
  Constant/1 -> Post Driver Intnded Axle Torque/6(Motor_Speed)

== system Milford/Controller_with_Transmission_Manager1/HSC/Powertrain Manager/HV Manager ==
  Sensors : Inport
  Controls : Inport  Port=2
  Axiomatic_Output_Manager : Subsystem
  BMS_Manager : Subsystem
  Bus Creator1 : BusCreator  Inputs=5
  DCDC Manager : Subsystem
  Inverter Manager : Subsystem
  OBC_Manager : Subsystem
  BMS_CAN : Outport
  HV_BUS_Status : Outport  Port=2
  OBC_CAN : Outport  Port=3
  OBC_Digital : Outport  Port=4
  BMS_Digital : Outport  Port=5
  Axiomatic_CAN : Outport  Port=6
  tag scope: MCU_CAN=global
  wires:
  Axiomatic_Output_Manager/1(Axiomatic_CAN) -> Axiomatic_CAN/1
  BMS_Manager/3(BMS Digital) -> BMS_Digital/1
  BMS_Manager/1(BMS CAN) -> BMS_CAN/1
  Controls/1 -> DCDC Manager/2(Control), Inverter Manager/3(Control), BMS_Manager/2(Controls)
  OBC_Manager/2(OBC_Digital) -> OBC_Digital/1
  OBC_Manager/1(OBC CAN) -> OBC_CAN/1
  [HV_BUS_Status] -> OBC_Manager/1(HV_Status)
  BMS_Manager/2(HV_BUS_Status) -> HV_BUS_Status/1  "HV_BUS_Status"
  [HV_BUS_Status] -> Axiomatic_Output_Manager/2(HV_Bus_Status)
  [HV_BUS_Status] -> Inverter Manager/1(HV_Bus_Status)  "HV_BUS_Status"
  Sensors/1 -> BMS_Manager/1(Sensors), OBC_Manager/2(Sensors), Axiomatic_Output_Manager/1(Sensors), DCDC Manager/1(BMSInput), Inverter Manager/2(Sensors)
  Inverter Manager/1(MCU_Status) -> Bus Creator1/1  "MCU_Status"
  Inverter Manager/2(MCU_CAN) -> Bus Creator1/2  "MCU_CAN"
  Inverter Manager/3(MCU_Torque_disconnect) -> Bus Creator1/3  "MCU_TorqueDscnt"
  Inverter Manager/4(MCU_Relay) -> Bus Creator1/4  "MCU_Relay"
  Bus Creator1/1 -> [MCU_CAN]
  DCDC Manager/1(DCDC_Status) -> Bus Creator1/5  "DCDC_Out"

== system Milford/Controller_with_Transmission_Manager1/HSC/Powertrain Manager/HV Manager1 ==
  Sensors : Inport
  Controls : Inport  Port=2
  Axiomatic_Output_Manager : Subsystem
  BMS_Manager : Subsystem
  DCDC Manager : Subsystem
  OBC_Manager : Subsystem
  BMS_CAN : Outport
  HV_BUS_Status : Outport  Port=2
  OBC_CAN : Outport  Port=3
  OBC_Digital : Outport  Port=4
  BMS_Digital : Outport  Port=5
  Axiomatic_CAN : Outport  Port=6
  Out1 : Outport  Port=7
  wires:
  [DCDC_Out] -> BMS_Manager/3(In1)
  DCDC Manager/1(Out1) -> Out1/1, [DCDC_Out]  "DCDC_Out"
  Sensors/1 -> BMS_Manager/1(Sensors), DCDC Manager/1(BMSInput), Axiomatic_Output_Manager/1(Sensors), OBC_Manager/2(Sensors)
  [HV_BUS_Status] -> Axiomatic_Output_Manager/2(HV_Bus_Status)
  BMS_Manager/2(HV_BUS_Status) -> [HV_BUS_Status], HV_BUS_Status/1  "HV_BUS_Status"
  [HV_BUS_Status] -> OBC_Manager/1(HV_Status)
  OBC_Manager/1(OBC CAN) -> OBC_CAN/1
  OBC_Manager/2(OBC_Digital) -> OBC_Digital/1
  Controls/1 -> BMS_Manager/2(Controls), DCDC Manager/2(In1), DCDC Manager/3(In2)
  BMS_Manager/1(BMS CAN) -> BMS_CAN/1
  BMS_Manager/3(BMS Digital) -> BMS_Digital/1
  Axiomatic_Output_Manager/1(Axiomatic_CAN) -> Axiomatic_CAN/1

== system Milford/Controller_with_Transmission_Manager1/HSC/Powertrain Manager/Output Conversion ==
  In1 : Inport
  In2 : Inport  Port=2
  In3 : Inport  Port=3
  In4 : Inport  Port=4
  In5 : Inport  Port=5
  In8 : Inport  Port=6
  In9 : Inport  Port=7
  In10 : Inport  Port=8
  In11 : Inport  Port=9
  Bus Creator : BusCreator  Inputs=14
  Bus Creator1 : BusCreator  Inputs=9
  Bus Selector2 : BusSelector  OutputSignals=powerMode,EnablePrplsn,ClutchEngage,EngAppReq,EngOnReq,MtrTrqCmd,EnableInverter,EngTrqCmd,HV_req,SysPwrMd_0_3,TransShftLvrPos,VehSpdAvgDrvn_kph,AccPos_Perc,SportsModeEnable
  Data Type Conversion{,2..3,5..13} (12 alike) : DataTypeConversion
  Memory : Memory
  Out1 : Outport
  wires:
  In10/1 -> Bus Creator1/8
  In9/1 -> Bus Creator1/7
  In8/1 -> Bus Creator1/6
  Memory/1 -> Data Type Conversion/1
  Data Type Conversion13/1 -> Bus Creator/13  "AccPos_Perc"
  Bus Selector2/13 -> Data Type Conversion13/1  "<AccPos_Perc>"
  Data Type Conversion12/1 -> Bus Creator/12  "VehSpdAvgDrvn_kph"
  Bus Selector2/12 -> Data Type Conversion12/1  "<VehSpdAvgDrvn_kph>"
  Data Type Conversion11/1 -> Bus Creator/11  "ShftLvrPos"
  Bus Selector2/11 -> Data Type Conversion11/1  "<TransShftLvrPos>"
  In5/1 -> Bus Creator1/5
  Bus Creator/1 -> Bus Creator1/4  "Controls"
  In3/1 -> Bus Creator1/3
  In2/1 -> Bus Creator1/2
  In1/1 -> Bus Creator1/1
  Bus Creator1/1 -> Out1/1
  Data Type Conversion5/1 -> Bus Creator/5  "EngOnReq"
  Data Type Conversion/1 -> Bus Creator/1  "powerMode"
  Data Type Conversion10/1 -> Bus Creator/10  "SysPwrMd"
  Data Type Conversion9/1 -> Bus Creator/9  "HV_req"
  Data Type Conversion8/1 -> Bus Creator/8  "EngTrqCmd"
  Data Type Conversion7/1 -> Bus Creator/7  "Inverter_Enable"
  Data Type Conversion6/1 -> Bus Creator/6  "Torque_Command"
  Bus Selector2/4 -> Bus Creator/4  "<EngAppReq>"
  Data Type Conversion3/1 -> Bus Creator/3  "ClutchEngage"
  Data Type Conversion2/1 -> Bus Creator/2  "EnablePrplsn"
  Bus Selector2/10 -> Data Type Conversion10/1  "<SysPwrMd_0_3>"
  Bus Selector2/9 -> Data Type Conversion9/1  "<HV_req>"
  Bus Selector2/8 -> Data Type Conversion8/1  "<EngTrqCmd>"
  Bus Selector2/7 -> Data Type Conversion7/1  "<EnableInverter>"
  Bus Selector2/6 -> Data Type Conversion6/1  "<MtrTrqCmd>"
  Bus Selector2/5 -> Data Type Conversion5/1  "<EngOnReq>"
  Bus Selector2/3 -> Data Type Conversion3/1  "<ClutchEngage>"
  Bus Selector2/2 -> Data Type Conversion2/1  "<EnablePrplsn>"
  Bus Selector2/1 -> Memory/1  "<powerMode>"
  In4/1 -> Bus Selector2/1
  In11/1 -> Bus Creator1/9
  Bus Selector2/14 -> Bus Creator/14  "<SportsModeEnable>"

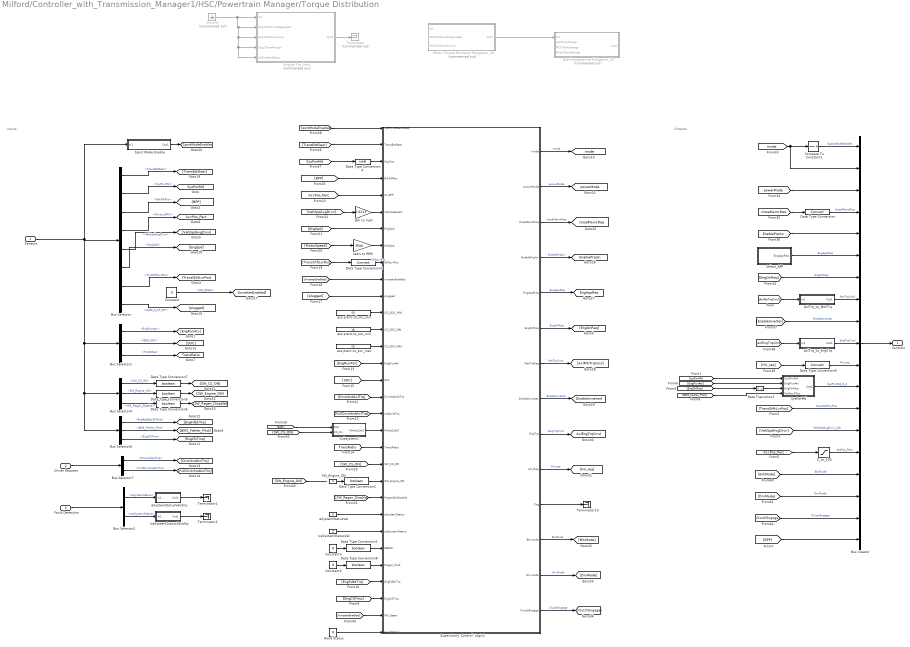
== system Milford/Controller_with_Transmission_Manager1/HSC/Powertrain Manager/Torque Distribution ==
  note: Outputs
  note: Inputs
  Sensors : Inport
  Driver Request : Inport  Port=2
  Fault Detection : Inport  Port=3
  0_to_100 : Saturate  UpperLimit=100  LowerLimit=0
  AxlTrq_to_EngTrq : Subsystem
  AxlTrq_to_MotTrq : Subsystem
  Bus Creator : BusCreator  Inputs=19
  Bus Selector : BusSelector  OutputSignals=from_CAN.fromVEH_CAN.from_TCM.TransEstGear,from_CAN.fromVEH_CAN.from_BCM.SysPwrMd,from_CAN.fromVEH_CAN.from_BCM.BrkPdlPos,from_Analog.Driver_APP1,from_CAN.fromEBCAN.from_ECM.VehSpdAvgDrvn,from_CAN.fromEBCAN.from_ECM.EngSpd,from_CAN.fromVEH_CAN.from_TCM.TrnsShftLvrPos,from_CAN.fromHV_CAN.from_OBC.NLG5_ST.NLG5_S_CP_DT
  Bus Selector1 : BusSelector  OutputSignals=from_CAN.fromEBCAN.from_ECM.EngRunAtv,from_CAN.fromHV_CAN.from_BMSHybrid.BMS_SOC,from_CAN.fromVEH_CAN.from_TCM.TrnGrRat
  Bus Selector2 : BusSelector  OutputSignals=eSystemDiagOut.eSystemStatus,iceSystemDiagOut.iceSystemStatus
  Bus Selector4 : BusSelector  OutputSignals=from_Digital.SW_CS_ON,from_Digital.SW_Engine_ON,from_Digital.SW_Regen_Disable
  Bus Selector6 : BusSelector  OutputSignals=from_CAN.fromEBCAN.from_ECM.EngActStdyStTorq,from_CAN.fromHV_CAN.from_BMSHybrid.BMS_HYB_02.BMS_Fehler_Pilot,from_CAN.fromEBCAN.from_ECM.EngCltTmp
  Bus Selector7 : BusSelector  OutputSignals=DrvIntndAxlTrq,FullDrvIntndAxlTrq
  Compare To Constant1 : simulink/Logic and Bit Operations/Compare To Constant  relop===  const=4  OutDataTypeStr=boolean
  Constant : Constant  Value=3
  Constant2 : Constant  Value=0
  Constant3 : Constant  Value=0
  Data Type Conversion : DataTypeConversion
  Data Type Conversion{1..2,5..8} (6 alike) : DataTypeConversion  OutDataTypeStr=boolean
  Data Type Conversion3 : DataTypeConversion
  Data Type Conversion4 : DataTypeConversion  OutDataTypeStr=int8
  Data Type Conversion9 : DataTypeConversion
  Engine Trq Limit : Subsystem  Commented=on
  Ground : Ground  Commented=on
  Hood Status : Constant  Value=0
  Motor Troque Mismatch Mitigation_CD : Subsystem  Commented=on
  OverTemperature Mitigation_CD : Subsystem  Commented=on
  Rate Transition3 : RateTransition
  SW_Engine_ON : Constant  Value=0
  Select_APP : Subsystem
  Sport Mode Enable : Subsystem
  Subsystem1 : Subsystem
  Supervisory  Control  Logic1 : Stateflow chart  TreatAsAtomicUnit=on
  SysPwrMd : Subsystem
  Terminator : Terminator  Commented=on
  Terminator1 : Terminator
  Terminator10 : Terminator
  Terminator2 : Terminator
  eSystemStatusVal : Constant  Value=0
  eSystemStatusValidity : Subsystem
  ess.plant.cd_soc_min : Constant  Value=50
  ess.plant.cs_soc_max : Constant  Value=23
  ess.plant.cs_soc_min : Constant  Value=18
  iceSystemStatusVal : Constant  Value=2
  iceSystemStatusValidity : Subsystem
  kph to mph : Gain  Gain=0.6213
  rad/s to RPM : Gain  Gain=30/pi
  Controls : Outport
  tag scope: AccPos_Perc=global, AxlEngTrqCmd=global, EnablePrplsn=global, EngAppReq=global, SportModeEnabled=global, SysPwrMd=global, TransRatio=global, closeMaincReq=global, mode=global, powerMode=global
  wires:
  [InverterEnabled] -> Supervisory  Control  Logic1/30(INV_State)
  Data Type Conversion2/1 -> Supervisory  Control  Logic1/22(SW_Engine_ON)
  SW_Engine_ON/1 -> Data Type Conversion2/1
  ess.plant.cd_soc_min/1 -> Supervisory  Control  Logic1/12(CD_SOC_MIN)
  ess.plant.cs_soc_min/1 -> Supervisory  Control  Logic1/13(CS_SOC_MIN)
  ess.plant.cs_soc_max/1 -> Supervisory  Control  Logic1/14(CS_SOC_MAX)
  Supervisory  Control  Logic1/8(EnableInverter) -> [EnableInverter]  "EnableInverter"
  Supervisory  Control  Logic1/4(EnablePrplsn) -> [EnablePrplsn]  "EnablePrplsn"
  Supervisory  Control  Logic1/3(closeMaincReq) -> [closeMaincReq]  "closeMaincReq"
  Supervisory  Control  Logic1/2(powerMode) -> [powerMode]  "powerMode"
  Supervisory  Control  Logic1/1(mode) -> [mode]  "mode"
  Data Type Conversion3/1 -> Supervisory  Control  Logic1/9(ShftLvrPos)  "ShftLvrPos"
  kph to mph/1 -> Supervisory  Control  Logic1/6(VehicleSpeed)
  Constant2/1 -> Data Type Conversion8/1
  Engine Trq Limit/1(Out1) -> Terminator/1
  Motor Troque Mismatch Mitigation_CD/1(Out1) -> OverTemperature Mitigation_CD/1(In1)
  Supervisory  Control  Logic1/11(Chg) -> Terminator10/1
  [DrvIntndAxlTrq] -> Supervisory  Control  Logic1/17(DrvIntdAxleTrq)
  [FullDrvIntndAxlTrq] -> Supervisory  Control  Logic1/18(IntdAxleTrq)
  Constant3/1 -> Data Type Conversion1/1
  Data Type Conversion1/1 -> Supervisory  Control  Logic1/26(ABSAtv)
  Subsystem1/1(Faked_SoC) -> Supervisory  Control  Logic1/19(Faked_SoC)
  Supervisory  Control  Logic1/12(Brkmode) -> [BrkMode]  "BrkMode"
  Data Type Conversion8/1 -> Supervisory  Control  Logic1/27(Regen_fault)
  iceSystemStatusVal/1 -> Supervisory  Control  Logic1/25(iceSystemStatus)
  eSystemStatusVal/1 -> Supervisory  Control  Logic1/24(eSystemStatus)
  Supervisory  Control  Logic1/5(EngAppReq) -> [EngAppReq]  "EngAppReq"
  rad/s to RPM/1 -> Supervisory  Control  Logic1/8(MotSpd)
  [EngCltTmp] -> Supervisory  Control  Logic1/29(EngCtlTmp)
  [EngFdbkTrq] -> Supervisory  Control  Logic1/28(EngFdbkTrq)
  [EngRunAtv] -> Supervisory  Control  Logic1/15(EngRunAtv)
  [TransRatio] -> Supervisory  Control  Logic1/20(TransRatio)
  [SOC] -> Supervisory  Control  Logic1/16(SoC)
  [SOC] -> Subsystem1/1(SoC)
  [InverterEnabled] -> Supervisory  Control  Logic1/10(InverterEnabled)
  [TransShftLvrPos] -> Data Type Conversion3/1
  [MotorSpeed] -> rad/s to RPM/1
  [EngSpd] -> Supervisory  Control  Logic1/7(EngSpd)
  [VehSpdAvgDrvn] -> kph to mph/1
  [AccPos_Perc] -> Supervisory  Control  Logic1/5(drvAPP)
  [BPP] -> Supervisory  Control  Logic1/4(BrkPdlPos)
  [TransEstGear] -> Supervisory  Control  Logic1/2(TransEstGear)
  [SysPwrMd] -> Data Type Conversion4/1
  Data Type Conversion4/1 -> Supervisory  Control  Logic1/3(KeyPos)
  [SportModeEnabled] -> Supervisory  Control  Logic1/1(SportModeEnabled)
  [SW_CS_ON] -> Supervisory  Control  Logic1/21(SW_CS_ON)
  [SW_Engine_ON] -> ?
  [SW_Regen_Disable] -> Supervisory  Control  Logic1/23(RegenBrkDisable)
  [SW_CS_ON] -> Subsystem1/2(CS_On)
  Supervisory  Control  Logic1/6(EngOnReq) -> [EngOnReq]  "EngOnReq"
  Supervisory  Control  Logic1/7(MotTrqReq) -> [AxlMtrTrqCmd]  "MtrTrqCmd"
  Supervisory  Control  Logic1/9(EngTrq) -> [AxlEngTrqCmd]  "EngTrqCmd"
  Supervisory  Control  Logic1/10(HV_Req) -> [HV_req]  "HV_req"
  Supervisory  Control  Logic1/13(Drvmode) -> [DrvMode]  "DrvMode"
  Supervisory  Control  Logic1/14(ClutchEngage) -> [ClutchEngage]  "ClutchEngage"
  Bus Selector7/1 -> [DrvIntndAxlTrq]  "<DrvIntndAxlTrq>"
  Driver Request/1 -> Bus Selector7/1
  Data Type Conversion7/1 -> [SW_CS_ON]
  Bus Selector1/2 -> [SOC]  "<BMS_SOC>"
  Sport Mode Enable/1(Out1) -> [SportModeEnabled]
  Bus Selector7/2 -> [FullDrvIntndAxlTrq]  "<FullDrvIntndAxlTrq>"
  Bus Selector6/3 -> [EngCltTmp]  "<EngCltTmp>"
  Bus Selector6/2 -> [BMS_Fehler_Pilot]  "<BMS_Fehler_Pilot>"
  Bus Selector6/1 -> [EngFdbkTrq]  "<EngActStdyStTorq>"
  Data Type Conversion6/1 -> [SW_Regen_Disable]
  Data Type Conversion5/1 -> [SW_Engine_ON]
  Bus Selector/8 -> [plugged]  "<NLG5_S_CP_DT>"
  iceSystemStatusValidity/1(Out1) -> Terminator2/1
  eSystemStatusValidity/1(Out1) -> Terminator1/1
  Bus Selector4/2 -> Data Type Conversion5/1  "<SW_Engine_ON>"
  Bus Selector4/1 -> Data Type Conversion7/1  "<SW_CS_ON>"
  Bus Selector4/3 -> Data Type Conversion6/1  "<SW_Regen_Disable>"
  Bus Selector2/2 -> iceSystemStatusValidity/1(In1)  "<iceSystemStatus>"
  Bus Selector2/1 -> eSystemStatusValidity/1(In1)  "<eSystemStatus>"
  Fault Detection/1 -> Bus Selector2/1
  Bus Selector1/3 -> [TransRatio]  "<TrnGrRat>"
  Bus Selector/7 -> [TransShftLvrPos]  "<TrnsShftLvrPos>"
  Bus Selector1/1 -> [EngRunAtv]  "<EngRunAtv>"
  Constant/1 -> [InverterEnabled]  "<INV_State>"
  Bus Selector/6 -> [EngSpd]  "<EngSpd>"
  Bus Selector/5 -> [VehSpdAvgDrvn]  "<VehSpdAvgDrvn>"
  Bus Selector/4 -> [AccPos_Perc]  "<Driver_APP1>"
  Bus Selector/3 -> [BPP]  "<BrkPdlPos>"
  Bus Selector/2 -> [SysPwrMd]  "<SysPwrMd>"
  Bus Selector/1 -> [TransEstGear]  "<TransEstGear>"
  Sensors/1 -> Bus Selector6/1, Bus Selector4/1, Bus Selector1/1, Sport Mode Enable/1(In1), Bus Selector/1
  Bus Creator/1 -> Controls/1
  Rate Transition3/1 -> SysPwrMd/3(EngOnReq)
  [EngOnReq] -> Rate Transition3/1
  Data Type Conversion/1 -> Bus Creator/4  "closeMaincReq"
  [powerMode] -> Bus Creator/3
  0_to_100/1 -> Bus Creator/15  "AccPos_Perc"
  AxlTrq_to_MotTrq/1(Out1) -> Bus Creator/8  "MtrTrqCmd"
  [BrkMode] -> Bus Creator/16  "BrkMode"
  Select_APP/1(EngAppReq) -> Bus Creator/6  "EngAppReq"
  [HV_req] -> Data Type Conversion9/1
  [EngOnReq] -> Bus Creator/7  "EngOnReq"
  [EnableInverter] -> Bus Creator/9  "EnableInverter"
  [AccPos_Perc] -> 0_to_100/1
  [EnablePrplsn] -> Bus Creator/5
  [BMS_Fehler_Pilot] -> SysPwrMd/4(Fehler_Pilot)
  Data Type Conversion9/1 -> Bus Creator/11  "HV_req"
  [VehSpdAvgDrvn] -> Bus Creator/14  "VehSpdAvgDrvn_kph"
  SysPwrMd/1(Out1) -> Bus Creator/12  "SysPwrMd_0_3"
  [SysPwrMd] -> SysPwrMd/1(SysPwrMd)
  [DrvMode] -> Bus Creator/17  "DrvMode"
  [TransShftLvrPos] -> Bus Creator/13  "TransShftLvrPos"
  [mode] -> Bus Creator/2, Compare To Constant1/1
  [AxlEngTrqCmd] -> AxlTrq_to_EngTrq/1(In1)
  [AxlMtrTrqCmd] -> AxlTrq_to_MotTrq/1(In1)
  [BPP] -> Bus Creator/19
  [ClutchEngage] -> Bus Creator/18  "ClutchEngage"
  [EngRunAtv] -> SysPwrMd/2(EngRunAtv)
  Compare To Constant1/1 -> Bus Creator/1  "SportsModeEnable"
  [closeMaincReq] -> Data Type Conversion/1
  AxlTrq_to_EngTrq/1(Out1) -> Bus Creator/10  "EngTrqCmd"
  [plugged] -> Supervisory  Control  Logic1/11(plugged)
  Ground/1 -> Engine Trq Limit/5(iceSystemStatus), Engine Trq Limit/4(Eng_TempRange), Engine Trq Limit/3(EngTrqMismchLimp), Engine Trq Limit/2(EngTrqMismchDegraded), Engine Trq Limit/1(In1)
  Hood Status/1 -> Supervisory  Control  Logic1/31(HoodStatus)

== system Milford/Sensors/CAN/EBCAN/BMS_Antrieb ==
  In1 : Inport
  Bus Creator : BusCreator  Inputs=2
  Bus Selector : BusSelector  OutputSignals=NMH_BMS,ISO_Hybrid_01_Resp
  ISO_Hybrid_01_Resp : Subsystem
  NMH_BMS : Subsystem
  Out1 : Outport
  wires:
  Bus Selector/2 -> ISO_Hybrid_01_Resp/1(In1)  "<ISO_Hybrid_01_Resp>"
  Bus Creator/1 -> Out1/1
  ISO_Hybrid_01_Resp/1(Out1) -> Bus Creator/2
  NMH_BMS/1(Out1) -> Bus Creator/1
  Bus Selector/1 -> NMH_BMS/1(In1)  "<NMH_BMS>"
  In1/1 -> Bus Selector/1

== system Milford/Sensors/CAN/EBCAN/CCM ==
  In1 : Inport
  Bus Creator : BusCreator  Inputs=2
  Bus Selector : BusSelector  OutputSignals=NMH_BMS,ISO_Hybrid_01_Resp
  ISO_Hybrid_01_Resp : Subsystem
  NMH_BMS : Subsystem
  Out1 : Outport
  wires:
  In1/1 -> Bus Selector/1
  Bus Selector/1 -> NMH_BMS/1(In1)  "<NMH_BMS>"
  NMH_BMS/1(Out1) -> Bus Creator/1
  ISO_Hybrid_01_Resp/1(Out1) -> Bus Creator/2
  Bus Creator/1 -> Out1/1
  Bus Selector/2 -> ISO_Hybrid_01_Resp/1(In1)  "<ISO_Hybrid_01_Resp>"
